simulink model "report_1_simulation"  (R2024a)
settings: Solver=VariableStepAuto  StartTime=0.0  StopTime=1000  RelTol=1e-3
settings Model: Creator=giuli  LastModifiedBy=giuli

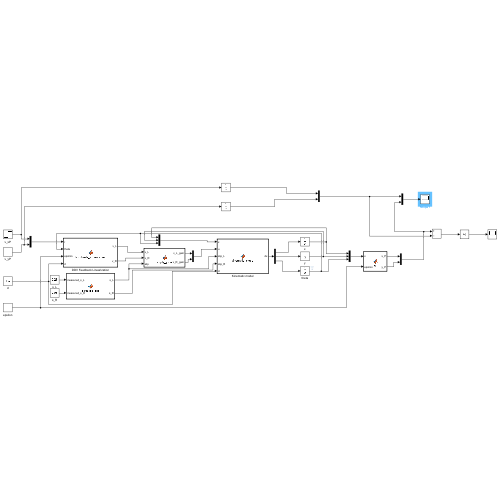
[thumbnail: Simulink's stored preview of the top-level diagram]
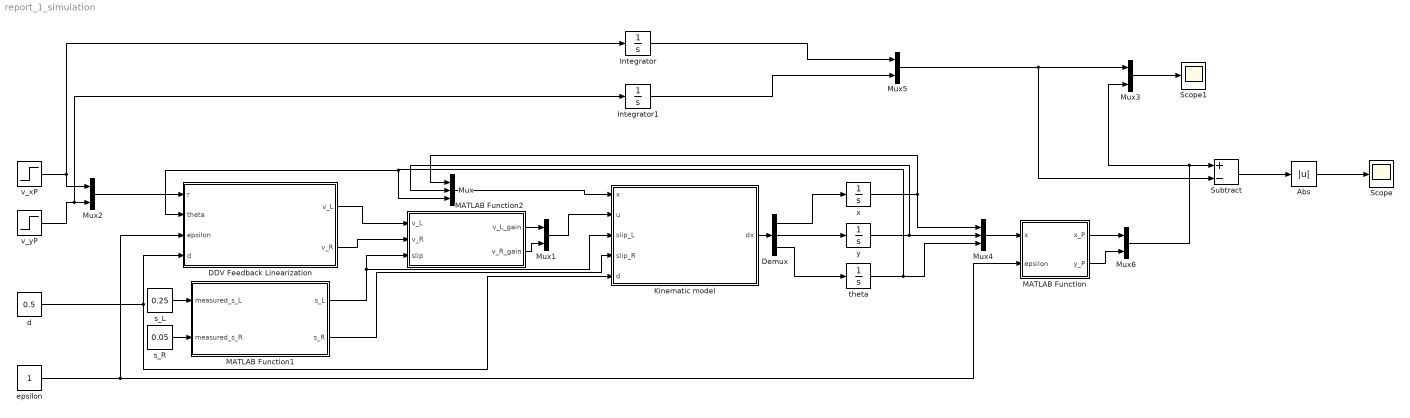
== system report_1_simulation ==
  Abs : Abs  SaturateOnIntegerOverflow=off
  DDV Feedback Linearization : MATLAB Function  TreatAsAtomicUnit=on
  Demux : Demux  Outputs=3
  Integrator : Integrator
  Integrator1 : Integrator
  Kinematic model : MATLAB Function  TreatAsAtomicUnit=on
  MATLAB Function : MATLAB Function  TreatAsAtomicUnit=on
  MATLAB Function1 : MATLAB Function  TreatAsAtomicUnit=on
  MATLAB Function2 : MATLAB Function  TreatAsAtomicUnit=on
  Mux : Mux  Inputs=3
  Mux{1..3,5..6} (5 alike) : Mux  Inputs=2
  Mux4 : Mux  Inputs=3
  Scope : Scope
  Scope1 : Scope
  Subtract : Sum  Inputs=+-
  d : Constant  Value=0.5
  epsilon : Constant
  s_L : Constant  Value=0.25
  s_R : Constant  Value=0.05
  theta : Integrator
  v_xP : Step  SampleTime=0
  v_yP : Step  Time=5  SampleTime=0
  x : Integrator
  y : Integrator
  wires:
  Kinematic model/1(dx) -> Demux/1
  Demux/1 -> x/1
  Demux/2 -> y/1
  Demux/3 -> theta/1
  x/1 -> Mux4/1, Mux/1
  y/1 -> Mux/2, Mux4/2
  theta/1 -> Mux4/3, DDV Feedback Linearization/2(theta), Mux/3
  Mux/1 -> Kinematic model/1(x)
  d/1 -> DDV Feedback Linearization/4(d), Kinematic model/5(d)
  Mux2/1 -> DDV Feedback Linearization/1(r)
  v_xP/1 -> Mux2/1, Integrator/1
  v_yP/1 -> Mux2/2, Integrator1/1
  epsilon/1 -> MATLAB Function/2(epsilon), DDV Feedback Linearization/3(epsilon)
  Mux4/1 -> MATLAB Function/1(x)
  Integrator/1 -> Mux5/1
  Integrator1/1 -> Mux5/2
  Mux5/1 -> Mux3/1, Subtract/2
  MATLAB Function/1(x_P) -> Mux6/1
  MATLAB Function/2(y_P) -> Mux6/2
  Mux6/1 -> Subtract/1, Mux3/2
  Subtract/1 -> Abs/1
  Abs/1 -> Scope/1
  MATLAB Function1/1(s_L) -> MATLAB Function2/3(slip), Kinematic model/3(slip_L)
  MATLAB Function1/2(s_R) -> Kinematic model/4(slip_R)
  s_R/1 -> MATLAB Function1/2(measured_s_R)
  s_L/1 -> MATLAB Function1/1(measured_s_L)
  DDV Feedback Linearization/2(v_R) -> MATLAB Function2/2(v_R)
  DDV Feedback Linearization/1(v_L) -> MATLAB Function2/1(v_L)
  Mux1/1 -> Kinematic model/2(u)
  MATLAB Function2/1(v_L_gain) -> Mux1/1
  MATLAB Function2/2(v_R_gain) -> Mux1/2
  Mux3/1 -> Scope1/1

== matlab function report_1_simulation/DDV Feedback Linearization ==
  data: r input; v_L output; theta input; epsilon input; d input; v_R output
function [v_L, v_R] = feedback_linearization(r, theta, epsilon, d)
    v_xP = r(1);
    v_yP = r(2);

    v_x = v_xP*cos(theta) + v_yP*sin(theta);
    omega = -1/epsilon*sin(theta)*v_xP + 1/epsilon*cos(theta)*v_yP;

    v_L = v_x - d*omega;
    v_R = v_x + d*omega;
end

== matlab function report_1_simulation/Kinematic model ==
  data: x input size=3; u input size=2; dx output size=3; slip_L input size=1; slip_R input size=1; d input
function dx  = kinematic_model(x, u, slip_L, slip_R, d)
    eta_L = 1-slip_L;
    eta_R = 1-slip_R;

    v_L = u(1);
    v_R = u(2);

    theta = x(3);

    dx = zeros(3,1);
    dx(1) = .5*eta_R*cos(theta)*v_R + .5*eta_L*cos(theta)*v_L;
    dx(2) = .5*eta_R*sin(theta)*v_R + .5*eta_L*sin(theta)*v_L;
    dx(3) = .5*(eta_R/d) - .5*(eta_L/d);
end

== matlab function report_1_simulation/MATLAB Function ==
  data: x input; x_P output; epsilon input; y_P output
function [x_P, y_P] = fl(x, epsilon)
    x_P = x(1) + epsilon*cos(x(3));
    y_P = x(2) + epsilon*sin(x(3));
end

== matlab function report_1_simulation/MATLAB Function1 ==
  data: measured_s_L input; s_L output; measured_s_R input; s_R output
function [s_L, s_R] = equalize_slip(measured_s_L, measured_s_R)
    avg_slip = (measured_s_L+measured_s_R) / 2;

    s_L = avg_slip;
    s_R = avg_slip;
end

== matlab function report_1_simulation/MATLAB Function2 ==
  data: v_L input; v_L_gain output; v_R input; slip input; v_R_gain output
function [v_L_gain, v_R_gain] = apply_gain(v_L, v_R, slip)
    eta = 1 - slip;
    gain = 1 / eta;
    
    v_L_gain = gain * v_L;
    v_R_gain = gain * v_R;
end
